simulink model "px4_controllers"  (R2018a)
settings: Solver=ode4  StartTime=0.0  StopTime=sim_time  FixedStep=1/sim_freq  MaxStep=0.0025  MinStep=0.0005  RelTol=1e-3
values from neighbouring files (symbols this model uses):
  C_D = [0.025; 0.025; 0.025]    [quad_parameters_IARTF.m]    (also in quad_parameters_SLADe.m = [0.5; 0.5; 0.5])
  d = 0.1275    [quad_parameters_IARTF.m]    (also in quad_parameters_SLADe.m = 0.465)
  eta_w = 0.2    [init_sim.m]
  euler_trim = zeros(3,1)    [controller_gains_IARTF.m]    (also in controller_gains_SLADe.m)
  g = 9.81    [init_sim.m]
  I = [Ixx 0 0 ; 0 Iyy 0 ; 0 0 Izz]    [init_sim.m]
  K_qd = (q_z1*q_z2)*K_qi    [controller_gains_SLADe.m]
  K_qi = 118.98/max_T    [controller_gains_SLADe.m]
  K_qp = (q_z1+q_z2)*K_qi    [controller_gains_SLADe.m]
  K_theta = K_theta_P + K_theta_I/s + K_theta_D*s    [controller_design_IARTF.m]    (also in controller_gains_SLADe.m = 9.1159)
  K_ud = (u_z1*u_z2)*K_ui    (= -0.0995091575092)    [controller_gains_SLADe.m]
  K_ui = -1.3583    [controller_gains_SLADe.m]
  K_up = (u_z1+u_z2)*K_ui    (= -0.769205787546)    [controller_gains_SLADe.m]
  m = 1.15    [quad_parameters_IARTF.m]    (also in quad_parameters_SLADe.m = 15)
  max_T = max_total_T / 4    [init_sim.m]
  ned_trim = zeros(3,1) + [0; 0; 0]    [controller_gains_IARTF.m]    (also in controller_gains_SLADe.m)
  PID_FILT_COEFF = 100    [controller_gains_IARTF.m]    (also in controller_gains_SLADe.m)
  pitch_rate_step_time = 0    [init_sim.m]
  pitch_rate_step_val = 0    [init_sim.m]
  pitch_step_time = 0    [init_sim.m]
  pitch_step_val = 0    [init_sim.m]
  q_int_lim = 0.3    [controller_gains_SLADe.m]
  r_D = 0.115*0.375    (= 0.043125)    [quad_parameters_IARTF.m]    (also in quad_parameters_SLADe.m = 0.18)
  R_LD = 10    [init_sim.m]
  rho = 1.225    [init_sim.m]
  T_trim = hover_T/4 * ones(4,1)    [controller_gains_IARTF.m]    (also in controller_gains_SLADe.m)
  tau_T = 0.05    [quad_parameters_IARTF.m]    (also in quad_parameters_SLADe.m = 0.125)
  vb_trim = zeros(3,1)    [controller_gains_IARTF.m]    (also in controller_gains_SLADe.m)
  virtual_controls_mat = [ 1,  1,  1,  1 ... (first row only)    [quad_parameters_IARTF.m]    (also in quad_parameters_SLADe.m = [1 1 1 1; 0 -1 0 1; 1 0 -1 0; -1 1 -1 1])
  vx_step_time = 0    [init_sim.m]
  vx_step_val = 0    [init_sim.m]
  wb_trim = zeros(3,1)    [controller_gains_IARTF.m]    (also in controller_gains_SLADe.m)
settings Model: Creator=Martin  LastModifiedBy=anton

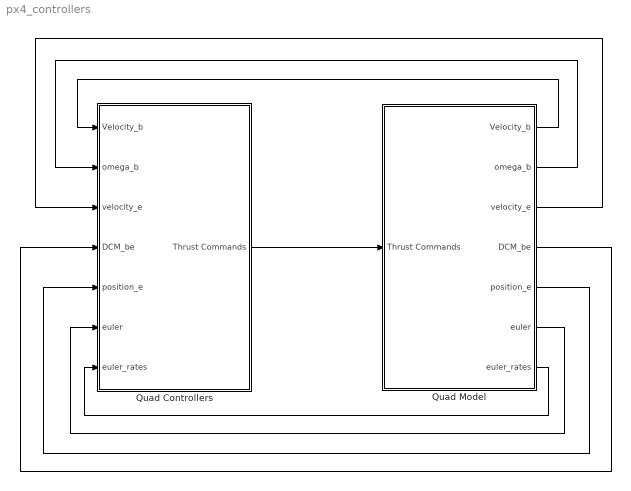
== system px4_controllers ==
  Quad Controllers : Subsystem  TreatAsAtomicUnit=on
  Quad Model : Subsystem  TreatAsAtomicUnit=on
  wires:
  Quad Controllers/1("Thrust Commands ") -> Quad Model/1(Thrust Commands)
  Quad Model/7("euler_rates ") -> Quad Controllers/7(euler_rates)
  Quad Model/6(euler) -> Quad Controllers/6(euler)
  Quad Model/5(position_e) -> Quad Controllers/5(position_e)
  Quad Model/4(DCM_be) -> Quad Controllers/4(DCM_be)
  Quad Model/1("Velocity_b ") -> Quad Controllers/1(Velocity_b)
  Quad Model/2(omega_b) -> Quad Controllers/2(omega_b)
  Quad Model/3(velocity_e) -> Quad Controllers/3(velocity_e)

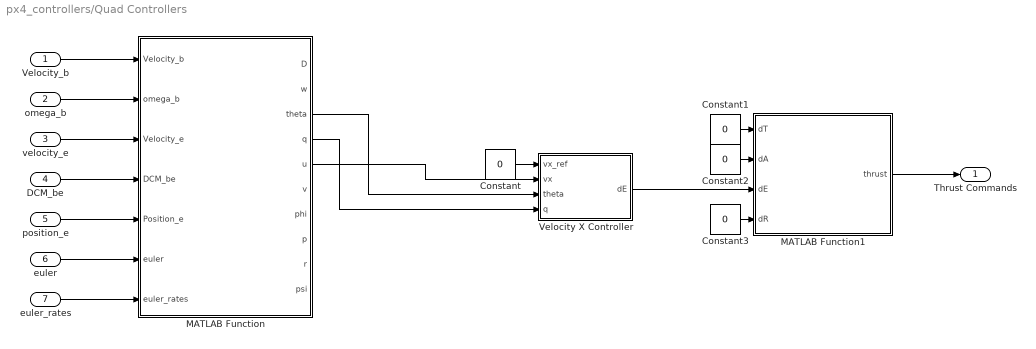
== system px4_controllers/Quad Controllers ==
  Velocity_b : Inport
  omega_b : Inport  Port=2
  velocity_e : Inport  Port=3
  DCM_be : Inport  Port=4
  position_e : Inport  Port=5
  euler : Inport  Port=6
  euler_rates : Inport  Port=7
  Constant{,1..3} (4 alike) : Constant  Value=0
  MATLAB Function : MATLAB Function  TreatAsAtomicUnit=on
  MATLAB Function1 : MATLAB Function  TreatAsAtomicUnit=on
  Velocity X Controller : Subsystem
  "Thrust Commands " : Outport
  wires:
  Velocity_b/1 -> MATLAB Function/1(Velocity_b)
  omega_b/1 -> MATLAB Function/2(omega_b)
  velocity_e/1 -> MATLAB Function/3(Velocity_e)
  DCM_be/1 -> MATLAB Function/4(DCM_be)
  position_e/1 -> MATLAB Function/5(Position_e)
  euler/1 -> MATLAB Function/6(euler)
  euler_rates/1 -> MATLAB Function/7(euler_rates)
  MATLAB Function1/1(thrust) -> "Thrust Commands "/1
  Constant1/1 -> MATLAB Function1/1(dT)
  Constant2/1 -> MATLAB Function1/2(dA)
  Constant3/1 -> MATLAB Function1/4(dR)
  Velocity X Controller/1(dE) -> MATLAB Function1/3(dE)
  MATLAB Function/5(u) -> Velocity X Controller/2(vx)
  MATLAB Function/3(theta) -> Velocity X Controller/3(theta)
  MATLAB Function/4(q) -> Velocity X Controller/4(q)
  Constant/1 -> Velocity X Controller/1(vx_ref)

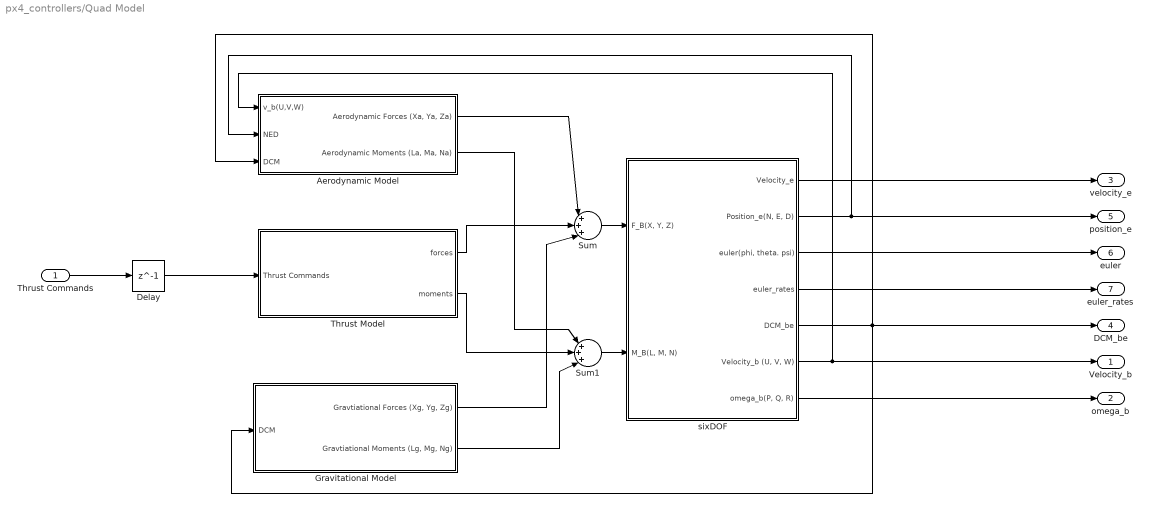
== system px4_controllers/Quad Model ==
  Thrust Commands : Inport
  Aerodynamic Model : Subsystem
  Delay : Delay  DelayLength=1
  Gravitational Model : Subsystem
  Sum : Sum  Inputs=|+++|
  Sum1 : Sum  Inputs=|+++|
  Thrust Model : Subsystem
  sixDOF : Subsystem
  "Velocity_b " : Outport
  omega_b : Outport  Port=2
  velocity_e : Outport  Port=3
  DCM_be : Outport  Port=4
  position_e : Outport  Port=5
  euler : Outport  Port=6
  "euler_rates " : Outport  Port=7
  wires:
  sixDOF/3("euler(phi, theta. psi)") -> euler/1
  sixDOF/5(DCM_be) -> Aerodynamic Model/3(DCM), DCM_be/1, Gravitational Model/1(DCM)
  Aerodynamic Model/2("Aerodynamic Moments (La, Ma, Na)") -> Sum1/1
  Thrust Commands/1 -> Delay/1
  Thrust Model/1(forces) -> Sum/2
  Sum1/1 -> sixDOF/2("M_B(L, M, N)")
  Thrust Model/2(moments) -> Sum1/2
  sixDOF/2("Position_e(N, E, D)") -> Aerodynamic Model/2(NED), position_e/1
  sixDOF/7("omega_b(P, Q, R)") -> omega_b/1
  Gravitational Model/2("Gravtiational Moments (Lg, Mg, Ng)") -> Sum1/3
  Gravitational Model/1("Gravtiational Forces (Xg, Yg, Zg)") -> Sum/3
  sixDOF/1(Velocity_e) -> velocity_e/1
  Aerodynamic Model/1("Aerodynamic Forces (Xa, Ya, Za)") -> Sum/1
  sixDOF/6("Velocity_b (U, V, W)") -> "Velocity_b "/1, Aerodynamic Model/1(v_b(U,V,W))
  Sum/1 -> sixDOF/1("F_B(X, Y, Z)")
  sixDOF/4(euler_rates) -> "euler_rates "/1
  Delay/1 -> Thrust Model/1(Thrust Commands)

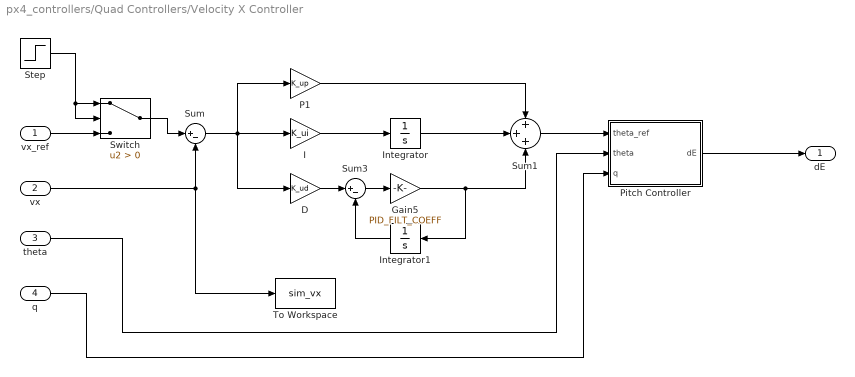
== system px4_controllers/Quad Controllers/Velocity X Controller ==
  vx_ref : Inport
  vx : Inport  Port=2
  theta : Inport  Port=3
  q : Inport  Port=4
  D : Gain  Gain=K_ud
  Gain5 : Gain  Gain=PID_FILT_COEFF
  I : Gain  Gain=K_ui
  Integrator : Integrator
  Integrator1 : Integrator
  P1 : Gain  Gain=K_up
  Pitch Controller : Subsystem
  Step : Step  Time=vx_step_time  After=vx_step_val  SampleTime=0
  Sum : Sum  Inputs=|+-
  Sum1 : Sum  Inputs=+++
  Sum3 : Sum  Inputs=|+-
  Switch : Switch  Criteria=u2 > Threshold
  To Workspace : ToWorkspace  VariableName=sim_vx  SaveFormat=Timeseries  SampleTime=-1
  dE : Outport
  wires:
  vx/1 -> To Workspace/1, Sum/2
  Pitch Controller/1(dE) -> dE/1
  Switch/1 -> Sum/1
  vx_ref/1 -> Switch/3
  Step/1 -> Switch/2, Switch/1
  I/1 -> Integrator/1
  Integrator1/1 -> Sum3/2
  P1/1 -> Sum1/1
  Sum3/1 -> Gain5/1
  Gain5/1 -> Sum1/3, Integrator1/1
  Sum1/1 -> Pitch Controller/1(theta_ref)
  Integrator/1 -> Sum1/2
  Sum/1 -> D/1, I/1, P1/1
  D/1 -> Sum3/1
  theta/1 -> Pitch Controller/2(theta)
  q/1 -> Pitch Controller/3(q)

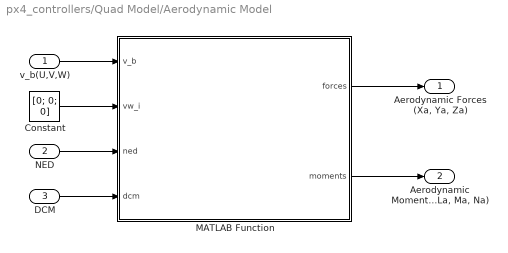
== system px4_controllers/Quad Model/Aerodynamic Model ==
  v_b(U,V,W) : Inport
  NED : Inport  Port=2
  DCM : Inport  Port=3
  Constant : Constant  Value=[0; 0; 0]
  MATLAB Function : MATLAB Function  TreatAsAtomicUnit=on
  "Aerodynamic Forces (Xa, Ya, Za)" : Outport
  "Aerodynamic Moments (La, Ma, Na)" : Outport  Port=2
  wires:
  MATLAB Function/1(forces) -> "Aerodynamic Forces (Xa, Ya, Za)"/1
  MATLAB Function/2(moments) -> "Aerodynamic Moments (La, Ma, Na)"/1
  v_b(U,V,W)/1 -> MATLAB Function/1(v_b)
  DCM/1 -> MATLAB Function/4(dcm)
  NED/1 -> MATLAB Function/3(ned)
  Constant/1 -> MATLAB Function/2(vw_i)

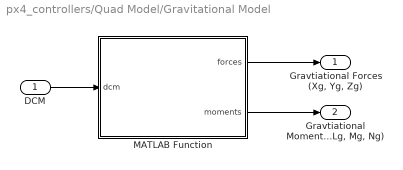
== system px4_controllers/Quad Model/Gravitational Model ==
  DCM : Inport
  MATLAB Function : MATLAB Function  TreatAsAtomicUnit=on
  "Gravtiational Forces (Xg, Yg, Zg)" : Outport
  "Gravtiational Moments (Lg, Mg, Ng)" : Outport  Port=2
  wires:
  DCM/1 -> MATLAB Function/1(dcm)
  MATLAB Function/1(forces) -> "Gravtiational Forces (Xg, Yg, Zg)"/1
  MATLAB Function/2(moments) -> "Gravtiational Moments (Lg, Mg, Ng)"/1

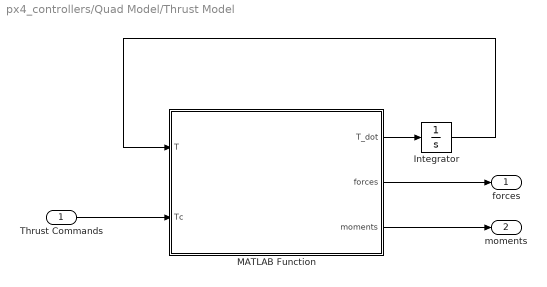
== system px4_controllers/Quad Model/Thrust Model ==
  Thrust Commands : Inport
  Integrator : Integrator  InitialCondition=T_trim
  MATLAB Function : MATLAB Function  TreatAsAtomicUnit=on
  forces : Outport
  moments : Outport  Port=2
  wires:
  Thrust Commands/1 -> MATLAB Function/2(Tc)
  MATLAB Function/1(T_dot) -> Integrator/1
  Integrator/1 -> MATLAB Function/1(T)
  MATLAB Function/2(forces) -> forces/1
  MATLAB Function/3(moments) -> moments/1

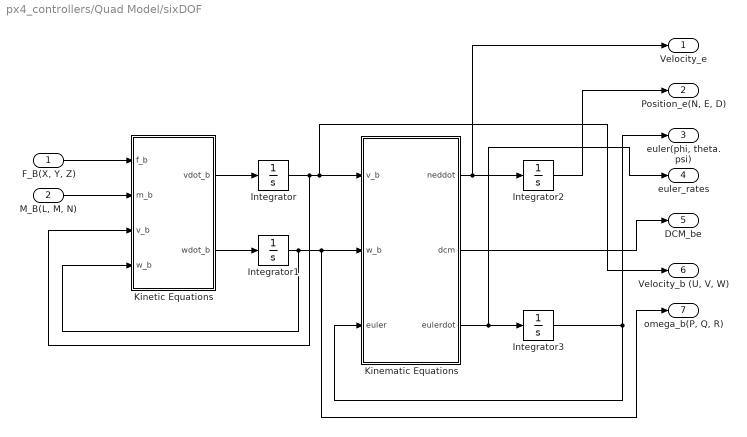
== system px4_controllers/Quad Model/sixDOF ==
  "F_B(X, Y, Z)" : Inport
  "M_B(L, M, N)" : Inport  Port=2
  Integrator : Integrator  InitialCondition=vb_trim
  Integrator1 : Integrator  InitialCondition=wb_trim
  Integrator2 : Integrator  InitialCondition=ned_trim
  Integrator3 : Integrator  InitialCondition=euler_trim  WrapState=on
  Kinematic Equations : MATLAB Function  TreatAsAtomicUnit=on
  Kinetic Equations : MATLAB Function  TreatAsAtomicUnit=on
  Velocity_e : Outport
  "Position_e(N, E, D)" : Outport  Port=2
  "euler(phi, theta. psi)" : Outport  Port=3
  euler_rates : Outport  Port=4
  DCM_be : Outport  Port=5
  "Velocity_b (U, V, W)" : Outport  Port=6
  "omega_b(P, Q, R)" : Outport  Port=7
  wires:
  "F_B(X, Y, Z)"/1 -> Kinetic Equations/1(f_b)
  "M_B(L, M, N)"/1 -> Kinetic Equations/2(m_b)
  Kinetic Equations/1(vdot_b) -> Integrator/1
  Kinetic Equations/2(wdot_b) -> Integrator1/1
  Integrator/1 -> Kinetic Equations/3(v_b), "Velocity_b (U, V, W)"/1, Kinematic Equations/1(v_b)
  Integrator1/1 -> Kinetic Equations/4(w_b), "omega_b(P, Q, R)"/1, Kinematic Equations/2(w_b)
  Kinematic Equations/2(dcm) -> DCM_be/1
  Kinematic Equations/3(eulerdot) -> Integrator3/1, euler_rates/1
  Kinematic Equations/1(neddot) -> Integrator2/1, Velocity_e/1
  Integrator2/1 -> "Position_e(N, E, D)"/1
  Integrator3/1 -> Kinematic Equations/3(euler), "euler(phi, theta. psi)"/1

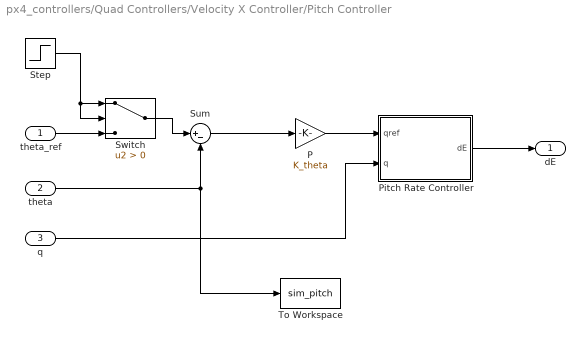
== system px4_controllers/Quad Controllers/Velocity X Controller/Pitch Controller ==
  theta_ref : Inport
  theta : Inport  Port=2
  q : Inport  Port=3
  P : Gain  Gain=K_theta
  Pitch Rate Controller : Subsystem
  Step : Step  Time=pitch_step_time  After=pitch_step_val  SampleTime=0
  Sum : Sum  Inputs=|+-
  Switch : Switch  Criteria=u2 > Threshold
  To Workspace : ToWorkspace  VariableName=sim_pitch  SaveFormat=Timeseries  SampleTime=-1
  dE : Outport
  wires:
  theta/1 -> To Workspace/1, Sum/2
  Sum/1 -> P/1
  P/1 -> Pitch Rate Controller/1(qref)
  q/1 -> Pitch Rate Controller/2(q)
  Pitch Rate Controller/1(dE) -> dE/1
  Switch/1 -> Sum/1
  theta_ref/1 -> Switch/3
  Step/1 -> Switch/2, Switch/1

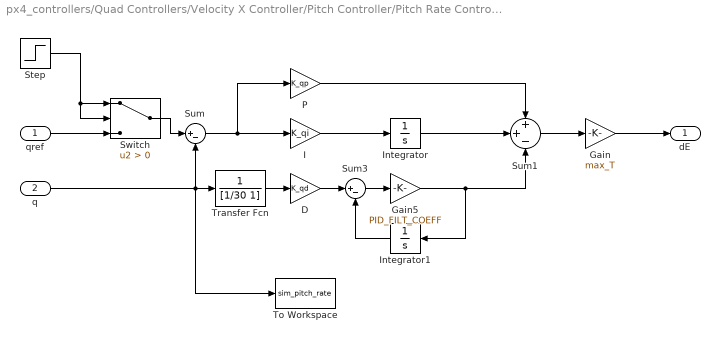
== system px4_controllers/Quad Controllers/Velocity X Controller/Pitch Controller/Pitch Rate Controller ==
  qref : Inport
  q : Inport  Port=2
  D : Gain  Gain=K_qd
  Gain : Gain  Gain=max_T
  Gain5 : Gain  Gain=PID_FILT_COEFF
  I : Gain  Gain=K_qi
  Integrator : Integrator  LimitOutput=on  UpperSaturationLimit=q_int_lim  LowerSaturationLimit=-0.3
  Integrator1 : Integrator
  P : Gain  Gain=K_qp
  Step : Step  Time=pitch_rate_step_time  After=pitch_rate_step_val  SampleTime=0
  Sum : Sum  Inputs=|+-
  Sum1 : Sum  Inputs=++-
  Sum3 : Sum  Inputs=|+-
  Switch : Switch  Criteria=u2 > Threshold
  To Workspace : ToWorkspace  VariableName=sim_pitch_rate  SaveFormat=Timeseries  SampleTime=-1
  Transfer Fcn : TransferFcn  Denominator=[1/30 1]
  dE : Outport
  wires:
  q/1 -> Transfer Fcn/1, To Workspace/1, Sum/2
  Sum/1 -> I/1, P/1
  I/1 -> Integrator/1
  Integrator1/1 -> Sum3/2
  Sum3/1 -> Gain5/1
  D/1 -> Sum3/1
  Gain5/1 -> Sum1/3, Integrator1/1
  P/1 -> Sum1/1
  Sum1/1 -> Gain/1
  Gain/1 -> dE/1
  Integrator/1 -> Sum1/2
  Switch/1 -> Sum/1
  qref/1 -> Switch/3
  Step/1 -> Switch/1, Switch/2
  Transfer Fcn/1 -> D/1

== matlab function px4_controllers/Quad Model/Aerodynamic Model/MATLAB Function ==
  data: v_b input size=3; vw_i input size=3; ned input size=3; dcm input size=[3,3]; rho parameter size=1; forces output size=3; moments output size=3; C_D parameter size=3; eta_w parameter size=1
function [forces, moments] = aerodynamicModel(v_b, vw_i, ned, dcm, rho, C_D, eta_w)
    
    vw_b = dcm * (power(abs(ned(3))/10, eta_w)) * vw_i;
    v_bw = -v_b + vw_b;
    q = 0.5 * rho * v_bw.*abs(v_bw);
    
    forces = q.*C_D;
    moments = [0; 0; 0];
    
end

== matlab function px4_controllers/Quad Controllers/MATLAB Function1 ==
  data: dT input; thrust output; dA input; dE input; dR input; mixin_mat parameter
function thrust = thrust_commands(dT, dA, dE, dR, mixin_mat)
    thrust = mixin_mat * [dT; dA; dE; dR];
end

== matlab function px4_controllers/Quad Model/Gravitational Model/MATLAB Function ==
  data: dcm input size=[3,3]; forces output size=3; moments output size=3; m parameter size=1; g parameter size=1
function [forces,moments] = gravitationalModel(dcm, m, g)

    moments = [0 ; 0 ; 0];
    forces = dcm * [0 ; 0 ; m*g];

end

== matlab function px4_controllers/Quad Model/Thrust Model/MATLAB Function ==
  data: T input size=4; T_dot output size=4; Tc input size=4; tau_T parameter size=1; forces output size=3; moments output size=3; d parameter size=1; r_D parameter size=1; virtual_controls_mat parameter size=[4,4]; R_LD parameter size=1
function [T_dot, forces, moments]  = thrustModel(T, Tc, tau_T, d, r_D, virtual_controls_mat, R_LD)

    virt_T = virtual_controls_mat * T;

    T_dot = (-T + Tc)/tau_T;
    forces = [0; 0; -virt_T(1)];
    moments = [d*virt_T(2); d*virt_T(3); r_D*virt_T(4)/R_LD];
    
end

== matlab function px4_controllers/Quad Model/sixDOF/Kinematic Equations ==
  data: v_b input size=3; w_b input size=3; euler input size=3; neddot output size=3; dcm output size=[3,3]; eulerdot output size=3
function [neddot, dcm, eulerdot] = kinematic(v_b, w_b, euler)
    phi = euler(1);
    theta = euler(2);
    psi = euler(3);

    eulerdot = [1 sin(phi)*tan(theta) cos(phi)*tan(theta) ; 0 cos(phi) -sin(phi) ; 0 sin(phi)/cos(theta) cos(phi)/cos(theta)] * w_b;

    euler3 = [1 0 0 ; 0 cos(phi) sin(phi) ; 0 -sin(phi) cos(phi)];
    euler2 = [cos(theta) 0 -sin(theta) ; 0 1 0 ; sin(psi) 0 cos(theta)];
    euler1 = [cos(psi) sin(psi) 0 ; -sin(psi) cos(psi) 0 ; 0 0 1];
    dcm = euler3 * euler2 * euler1;

    neddot = dcm' * v_b;
end

== matlab function px4_controllers/Quad Model/sixDOF/Kinetic Equations ==
  data: f_b input size=3; vdot_b output size=3; m_b input size=3; v_b input size=3; w_b input size=3; wdot_b output size=3; m parameter size=1; I parameter size=[3,3]
function [vdot_b, wdot_b] = kinetic(f_b, m_b, v_b, w_b, m, I)

    vdot_b = (f_b - cross(w_b, m*v_b))/m;
    wdot_b = I\(m_b - cross(w_b, I * w_b));
    
end

== matlab function px4_controllers/Quad Controllers/MATLAB Function ==
  data: Velocity_b input size=3; omega_b input size=3; Velocity_e input size=3; DCM_be input size=[3,3]; Position_e input size=3; euler input size=3; D output; euler_rates input size=3; w output; theta output; q output; u output; v output; phi output; p output; r output; psi output
function [D, w, theta, q, u, v, phi, p, r, psi] = fcn(Velocity_b, omega_b, Velocity_e, DCM_be, Position_e, euler, euler_rates)
    u = Velocity_b(1);
    v = Velocity_b(2);
    w = Velocity_b(3);
    
    p = omega_b(1);
    q = omega_b(2);
    r = omega_b(3);
    
    D = Position_e(3);
    
    phi = euler(1);
    theta = euler(2);
    psi = euler(3);
end
